simulink model "TestTriggerSubsystem"  (R2022a)
settings: Solver=VariableStepAuto  StartTime=0.0  StopTime=10.0  RelTol=1e-3
libraries: simulink x1
settings Model: Creator=tyevans  LastModifiedBy=tyevans

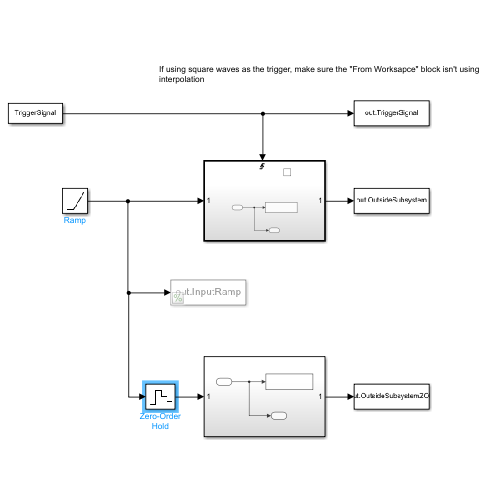
[thumbnail: Simulink's stored preview of the top-level diagram]
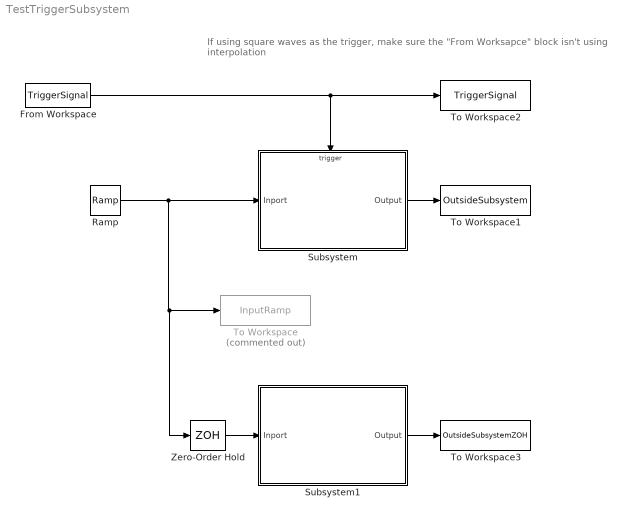
== system TestTriggerSubsystem ==
  note: If using square waves as the trigger, make sure the "From Worksapce" block isn't using interpolation
  From Workspace : FromWorkspace  VariableName=TriggerSignal  Interpolate=off  OutputAfterFinalValue=Holding final value
  Ramp : simulink/Sources/Ramp  slope=2  start=0  InitialOutput=0
  Subsystem : Subsystem
  Subsystem1 : Subsystem
  To Workspace : ToWorkspace  Commented=on  VariableName=InputRamp  SaveFormat=Timeseries  SampleTime=1/10
  To Workspace1 : ToWorkspace  VariableName=OutsideSubsystem  SaveFormat=Timeseries  SampleTime=-1
  To Workspace2 : ToWorkspace  VariableName=TriggerSignal  SaveFormat=Timeseries  SampleTime=-1
  To Workspace3 : ToWorkspace  VariableName=OutsideSubsystemZOH  SaveFormat=Timeseries  SampleTime=-1
  Zero-Order Hold : ZeroOrderHold  SampleTime=2
  wires:
  Ramp/1 -> Zero-Order Hold/1, To Workspace/1, Subsystem/1(Inport)
  From Workspace/1 -> Subsystem/Trigger, To Workspace2/1
  Subsystem/1(Output) -> To Workspace1/1
  Subsystem1/1(Output) -> To Workspace3/1
  Zero-Order Hold/1 -> Subsystem1/1(Inport)

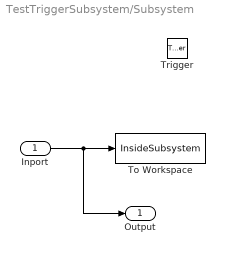
== system TestTriggerSubsystem/Subsystem ==
  Inport : Inport
  Trigger : TriggerPort  VariantControl=(inherit)  PortDimensions=1
  To Workspace : ToWorkspace  VariableName=InsideSubsystem  SaveFormat=Timeseries  SampleTime=-1
  Output : Outport
  wires:
  Inport/1 -> Output/1, To Workspace/1

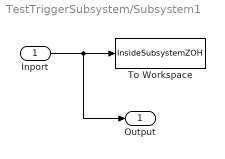
== system TestTriggerSubsystem/Subsystem1 ==
  Inport : Inport
  To Workspace : ToWorkspace  VariableName=InsideSubsystemZOH  SaveFormat=Timeseries  SampleTime=-1
  Output : Outport
  wires:
  Inport/1 -> Output/1, To Workspace/1
